simulink model "FW_formation_control_wind"  (R2023b)
settings: Solver=FixedStepAuto  StartTime=0.0  StopTime=70  FixedStep=0.001  RelTol=1e-3
undefined symbols (not defined in the file or in its folder): C, com, fc, hc, init, L, L2, lc, leader, tau, Va_max, Va_min
libraries: Fixed_Wing x3, simulink x1
(part 2 of 2)

== matlab function FW_formation_control_wind/Formation Controller/Lyapunov formation controller ==
  data: Va_Fc output size=1; G_desired input; G_error input; course_L input; course_L_dot input; z_L_dot input; V_L input; C input; Va_Fd output size=1; theta_Fc output size=1; theta_Fd output size=1; psi_Fc output size=1; Va_F input; psi_F input; theta_F input; tau input; psi_Fd output size=1
function [Va_Fc, Va_Fd,theta_Fc, theta_Fd,psi_Fc,psi_Fd ] = lyapunov_formation(G_desired, G_error, course_L, course_L_dot, z_L_dot, V_L, C, Va_F, psi_F ,theta_F, tau)
    lc = G_desired(1);
    fc = G_desired(2);
    hc = G_desired(3);
    le = G_error(1);
    fe = G_error(2);
    he = G_error(3);
    c1 = C(1);
    c2 = C(2);
    c3 = C(3);
    c4 = C(4);
    c5 = C(5);
    c6 = C(6);

    % course_F = atan2(-c1*le-course_L_dot*(fe+fc), c2*fe-course_L_dot*(le+lc)+V_L)+course_L;
    % V_F = sqrt((c1*le+course_L_dot*(fe+fc))^2+(c2*fe-course_L_dot*(le+lc)+V_L)^2);

    psi_Fd = atan2(-c1*le-course_L_dot*fc, c2*fe-course_L_dot*lc+V_L)+course_L;
    Va_Fd = sqrt((c1*le+course_L_dot*fc)^2+(c2*fe-course_L_dot*lc+V_L)^2);
    
    % ensure that the value in asin funtion fall between [-1,1]
    c = c3*he-z_L_dot;
    if c > Va_Fd
        c = Va_Fd;
    elseif c < -Va_Fd
        c = -Va_Fd;
    end

    theta_Fd = asin(c/Va_Fd);

    V_L_dot = 0;
    Va_Fe = Va_F-Va_Fd;
    psie = psi_F-psi_Fd;
    theta_Fe = theta_F-theta_Fd;
    
    alpha = tau(1);
    beta = tau(2);
    gamma = tau(3);

    le_dot = Va_F*sin(psi_F-course_L)+course_L_dot*(fe+fc);
    fe_dot = V_L-Va_F*cos(psi_F-course_L)-course_L_dot*(le+lc);
    he_dot = -z_L_dot-Va_F*sin(theta_F);

    a = -c1*le-course_L_dot*fc;
    a_dot = -c1*le_dot;
    b = c2*fe-course_L_dot*lc+V_L;
    b_dot = c2*fe_dot+V_L_dot;
    % c = c3*he-z_L_dot;
    c_dot = c3*he_dot;

    Va_Fc = 1/alpha*((a_dot*a+b*b_dot)/sqrt(a^2+b^2)-c4*Va_Fe)+Va_F;
    psi_Fc = 1/beta*((a_dot*b-a*b_dot)/(a^2+b^2)+course_L_dot-c5*psie)+psi_F;
    theta_Fc = 1/gamma*((c_dot*Va_Fd-c*((a_dot*a+b*b_dot)/sqrt(a^2+b^2)))/(Va_Fd*sqrt(Va_Fd^2-c^2))-c6*theta_Fe)+theta_F;

end
